simulink model "MBD_ques4"  (R2020a)
settings: Solver=FixedStepDiscrete  StartTime=0.0  StopTime=20  RelTol=1e-3
settings Model: Creator=DELL  LastModifiedBy=DELL

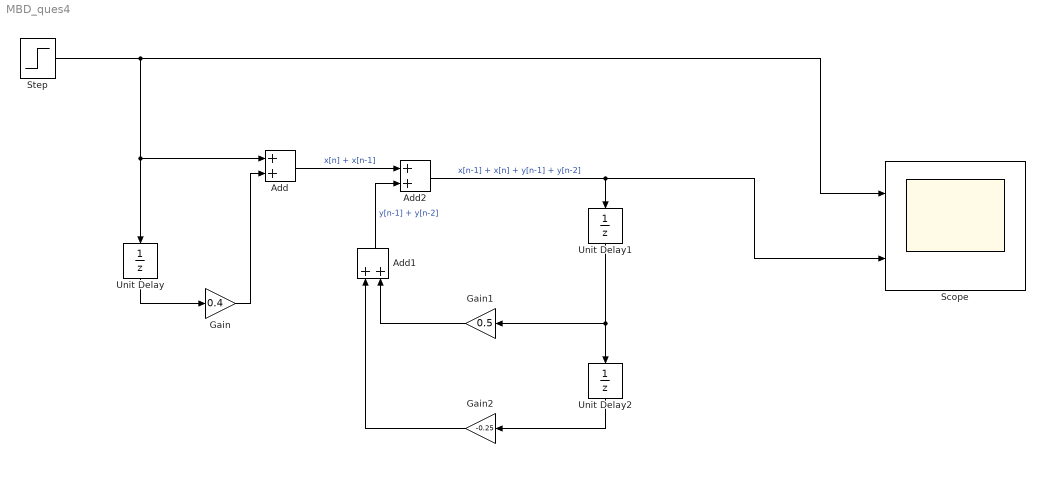
== system MBD_ques4 ==
  Add : Sum
  Add1 : Sum
  Add2 : Sum
  Gain : Gain  Gain=0.4
  Gain1 : Gain  Gain=0.5
  Gain2 : Gain  Gain=-0.25
  Scope : Scope  NumInputPorts=2
  Step : Step  SampleTime=0
  Unit Delay : UnitDelay  SampleTime=-1  HasFrameUpgradeWarning=on
  Unit Delay1 : UnitDelay  SampleTime=-1  HasFrameUpgradeWarning=on
  Unit Delay2 : UnitDelay  SampleTime=-1  HasFrameUpgradeWarning=on
  wires:
  Step/1 -> Unit Delay/1, Add/1, Scope/1
  Unit Delay/1 -> Gain/1
  Gain/1 -> Add/2
  Unit Delay1/1 -> Gain1/1, Unit Delay2/1
  Unit Delay2/1 -> Gain2/1
  Gain1/1 -> Add1/2
  Gain2/1 -> Add1/1
  Add1/1 -> Add2/2  "y[n-1] + y[n-2]"
  Add/1 -> Add2/1  "x[n] + x[n-1]"
  Add2/1 -> Scope/2, Unit Delay1/1  "x[n-1] + x[n] + y[n-1] + y[n-2]"
